simulink model "FG-fdm"  (R2022a)
settings: Solver=FixedStepAuto  StartTime=0.0  StopTime=Tend  FixedStep=Ts  MaxStep=0.033333333333333333  RelTol=1e-3
undefined symbols (not defined in the file or in its folder): A, B, C, D, Earth, h0, Ts, u0, v0, w0, WGS84, x0
libraries: aerolibconvert2 x3, aerolibfltsims x2, aerolibanimutils x1, aerolibtransform2 x1
settings Model: Creator=OSU  LastModifiedBy=Nick
settings DebuggingCC: UnconnectedInputMsg=warning  UnconnectedOutputMsg=warning  UnconnectedLineMsg=warning
settings RTWCC: DLArmComputeVersion=19.05

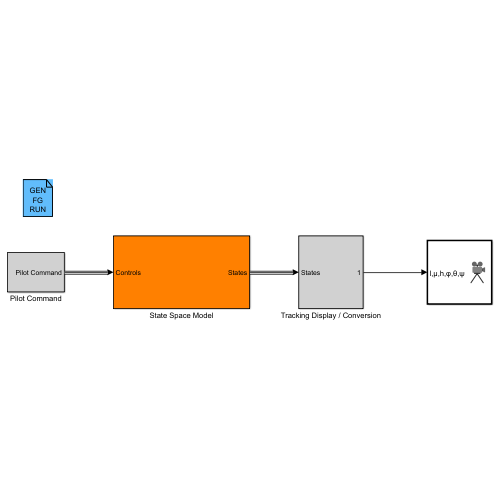
[thumbnail: Simulink's stored preview of the top-level diagram]
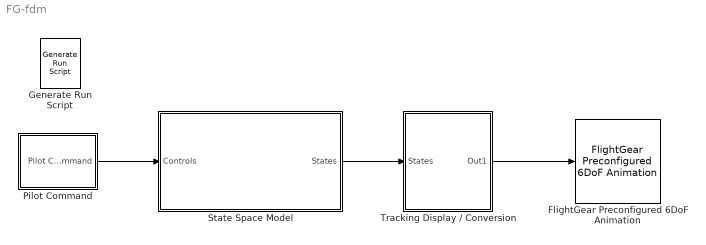
== system FG-fdm ==
  FlightGear Preconfigured 6DoF Animation : aerolibfltsims/FlightGear Preconfigured 6DoF Animation  xFlightGearVersion=v2019.1  DestinationIpAddress=127.0.0.1  DestinationPort=5502  SampleTime=Ts  packetVersion=24
  Generate Run Script : aerolibfltsims/Generate Run Script  Architecture=Default  dataFlow=Send  GeometryModelName=c172p_slx  AirportId=KSWO  RunwayId=35  InitialAltitude=5000  InitialHeading=0  OffsetDistance=0  OffsetAzimuth=0  InstallScenery=on  DisableShaders=off  OriginAddress=127.0.0.1  DestinationPort=5502  OriginPort=5505  LocalAddress=127.0.0.1  OutputFileName=runfg172p.bat  FlightGearBaseDirectory=C:\Program Files\FlightGear
  Pilot Command : Subsystem
  State Space Model : Subsystem
  Tracking Display / Conversion : Subsystem
  wires:
  Tracking Display / Conversion/1(Out1) -> FlightGear Preconfigured 6DoF Animation/1
  State Space Model/1(States) -> Tracking Display / Conversion/1(States)
  Pilot Command/1(Pilot Command) -> State Space Model/1(Controls)

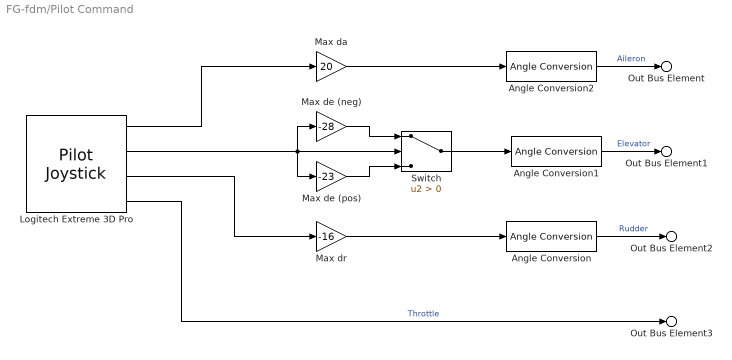
== system FG-fdm/Pilot Command ==
  Angle Conversion : aerolibconvert2/Angle Conversion  IU=deg  OU=rad
  Angle Conversion1 : aerolibconvert2/Angle Conversion  IU=deg  OU=rad
  Angle Conversion2 : aerolibconvert2/Angle Conversion  IU=deg  OU=rad
  Logitech Extreme 3D Pro : aerolibanimutils/Pilot Joystick  JoystickID=Joystick1  OutputConfiguration=FourAxis  SampleTime=Ts
  Max da : Gain  Gain=20
  Max de (neg) : Gain  Gain=-28
  Max de (pos) : Gain  Gain=-23
  Max dr : Gain  Gain=-16
  Switch : Switch  Criteria=u2 > Threshold  SaturateOnIntegerOverflow=off  InputSameDT=off
  Out Bus Element1 : Outport  PortName=Pilot Command  Element=Elevator
  Out Bus Element3 : Outport  PortName=Pilot Command  Element=Throttle
  Out Bus Element : Outport  PortName=Pilot Command  Element=Aileron
  Out Bus Element2 : Outport  PortName=Pilot Command  Element=Rudder
  wires:
  Logitech Extreme 3D Pro/3 -> Max dr/1
  Logitech Extreme 3D Pro/4 -> Out Bus Element3/1  "Throttle"
  Logitech Extreme 3D Pro/2 -> Max de (neg)/1, Max de (pos)/1, Switch/2
  Max de (neg)/1 -> Switch/1
  Max de (pos)/1 -> Switch/3
  Logitech Extreme 3D Pro/1 -> Max da/1
  Switch/1 -> Angle Conversion1/1
  Max da/1 -> Angle Conversion2/1
  Max dr/1 -> Angle Conversion/1
  Angle Conversion2/1 -> Out Bus Element/1  "Aileron"
  Angle Conversion1/1 -> Out Bus Element1/1  "Elevator"
  Angle Conversion/1 -> Out Bus Element2/1  "Rudder"

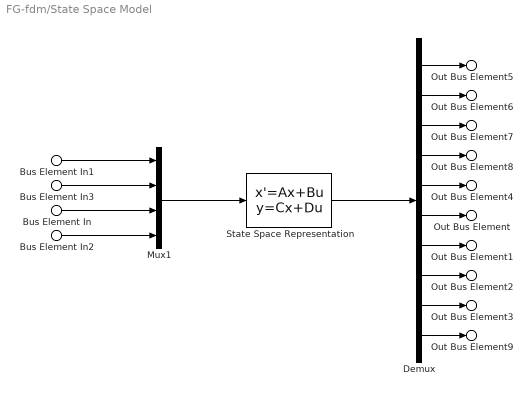
== system FG-fdm/State Space Model ==
  Bus Element In : Inport  PortName=Controls  Element=Aileron
  Bus Element In1 : Inport  PortName=Controls  Element=Elevator
  Bus Element In2 : Inport  PortName=Controls  Element=Rudder
  Bus Element In3 : Inport  PortName=Controls  Element=Throttle
  Demux : Demux  Outputs=10
  Mux1 : Mux
  State Space Representation : StateSpace  A=A  B=B  C=C  D=D  InitialCondition=x0
  Out Bus Element5 : Outport  PortName=States  Element=u
  Out Bus Element6 : Outport  PortName=States  Element=w
  Out Bus Element7 : Outport  PortName=States  Element=q
  Out Bus Element8 : Outport  PortName=States  Element=theta
  Out Bus Element : Outport  PortName=States  Element=v
  Out Bus Element1 : Outport  PortName=States  Element=p
  Out Bus Element2 : Outport  PortName=States  Element=r
  Out Bus Element3 : Outport  PortName=States  Element=phi
  Out Bus Element4 : Outport  PortName=States  Element=h
  Out Bus Element9 : Outport  PortName=States  Element=psi
  wires:
  Bus Element In/1 -> Mux1/3
  Bus Element In2/1 -> Mux1/4
  State Space Representation/1 -> Demux/1
  Demux/1 -> Out Bus Element5/1
  Demux/2 -> Out Bus Element6/1
  Demux/3 -> Out Bus Element7/1
  Demux/4 -> Out Bus Element8/1
  Bus Element In3/1 -> Mux1/2
  Mux1/1 -> State Space Representation/1
  Demux/5 -> Out Bus Element4/1
  Demux/6 -> Out Bus Element/1
  Demux/7 -> Out Bus Element1/1
  Demux/8 -> Out Bus Element2/1
  Demux/9 -> Out Bus Element3/1
  Demux/10 -> Out Bus Element9/1
  Bus Element In1/1 -> Mux1/1

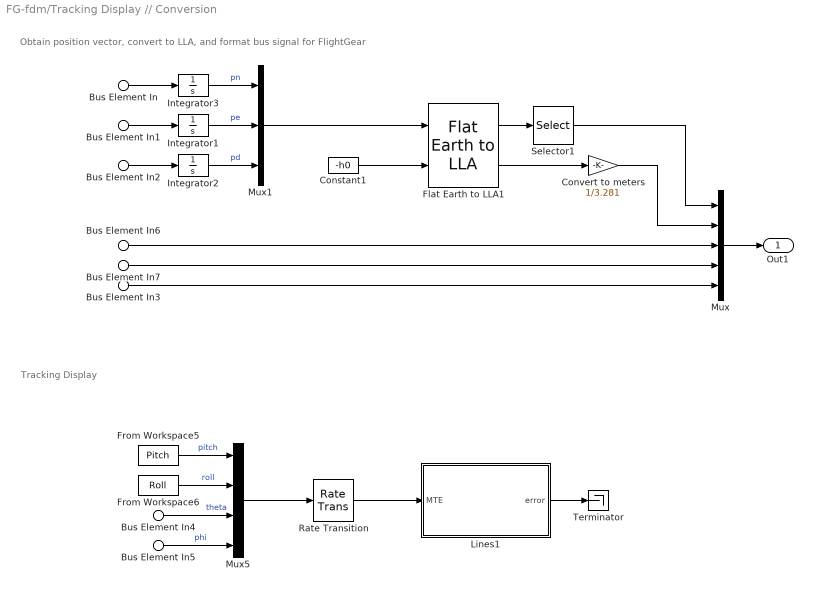
== system FG-fdm/Tracking Display // Conversion ==
  note: Tracking Display
  note: Obtain position vector, convert to LLA, and format bus signal for FlightGear
  Bus Element In : Inport  PortName=States  Element=u
  Bus Element In1 : Inport  PortName=States  Element=v
  Bus Element In2 : Inport  PortName=States  Element=w
  Bus Element In6 : Inport  PortName=States  Element=phi
  Bus Element In5 : Inport  PortName=States  Element=phi
  Bus Element In7 : Inport  PortName=States  Element=theta
  Bus Element In4 : Inport  PortName=States  Element=theta
  Bus Element In3 : Inport  PortName=States  Element=psi
  Constant1 : Constant  Value=-h0  SampleTime=Ts
  Convert to meters : Gain  Gain=1/3.281
  Flat Earth to LLA1 : aerolibtransform2/Flat Earth to LLA  units=English  ptype=Earth (WGS84)  F=1/298.257223563  R=20925646.3255  refPosPort=off  LL0=l_mu0  psi=0
  From Workspace5 : FromWorkspace  VariableName=Pitch  SampleTime=Ts  OutputAfterFinalValue=Setting to zero
  From Workspace6 : FromWorkspace  VariableName=Roll  SampleTime=Ts  OutputAfterFinalValue=Setting to zero
  Integrator1 : Integrator  InitialCondition=v0  ContinuousStateAttributes='v'
  Integrator2 : Integrator  InitialCondition=w0  ContinuousStateAttributes='w'
  Integrator3 : Integrator  InitialCondition=u0  ContinuousStateAttributes='u'
  Lines1 : MATLAB Function  TreatAsAtomicUnit=on
  Mux : Mux  Inputs=5
  Mux1 : Mux  Inputs=3
  Mux5 : Mux
  Rate Transition : RateTransition  OutPortSampleTimeOpt=Inherit  OutPortSampleTimeMultiple=2
  Selector1 : Selector  IndexMode=Zero-based  InputPortWidth=2  IndexOptions=Index vector (dialog)  Indices=[1 0]  OutputSizes=1
  Terminator : Terminator
  Out1 : Outport
  wires:
  Flat Earth to LLA1/1 -> Selector1/1
  Flat Earth to LLA1/2 -> Convert to meters/1
  Selector1/1 -> Mux/1
  Mux/1 -> Out1/1
  Bus Element In/1 -> Integrator3/1
  Bus Element In1/1 -> Integrator1/1
  Bus Element In6/1 -> Mux/3
  Bus Element In7/1 -> Mux/4
  Mux1/1 -> Flat Earth to LLA1/1
  Integrator1/1 -> Mux1/2  "pe"
  Integrator3/1 -> Mux1/1  "pn"
  Bus Element In2/1 -> Integrator2/1
  Bus Element In3/1 -> Mux/5
  Constant1/1 -> Flat Earth to LLA1/2
  Convert to meters/1 -> Mux/2
  Integrator2/1 -> Mux1/3  "pd"
  Bus Element In5/1 -> Mux5/4  "phi"
  Bus Element In4/1 -> Mux5/3  "theta"
  From Workspace6/1 -> Mux5/2  "roll"
  Mux5/1 -> Rate Transition/1
  From Workspace5/1 -> Mux5/1  "pitch"
  Lines1/1(error) -> Terminator/1
  Rate Transition/1 -> Lines1/1(MTE)

== matlab function FG-fdm/Tracking Display // Conversion/Lines1 ==
  data: MTE input; error output
function error = Display(MTE)

clf  % clear last frame

%-- Inputs --%
tht = MTE(1);
phi = MTE(2)*pi/180;
tht_x = MTE(3)*180/pi;
phi_x = MTE(4);

%-- Error signal output
error = [tht - tht_x; phi - phi_x];

%-- Transformation matrices --%
% MTE signal
R = [ cos(phi)  sin(phi)  0    ; 
     -sin(phi)  cos(phi) tht   ;
      0         0         1    ; ];
  
% Tolerance symbology
Rt = [ cos(phi_x)  sin(phi_x)  0     ;
      -sin(phi_x)  cos(phi_x)  tht_x ;
       0           0           1     ;];
   
    %% Calculate MTE signal and tolerance symbology orientation
        
%-- MTE signal line vector --%
% Transform vector coordinates
x0r = R * [ 10; 0; 1];     
x0l = R * [-10; 0; 1];

n = 25;     % for linspace()

% Transformed vector data for plotting
X = linspace(x0l(1), x0r(1), n);
Y = linspace(x0l(2), x0r(2), n);

%-- Tolerance vectors --%

% PITCH
rd = 1;     % Desired:  +/- 1 deg
ra = 2;     % Adequate: +/- 2 deg

ang = 0:0.01:2*pi;

xpd = rd*cos(ang);
ypd = rd*sin(ang);
xpa = ra*cos(ang);
ypa = ra*sin(ang);

N = ones(size(xpd));

Pd = Rt * [xpd; ypd; N];
Pa = Rt * [xpa; ypa; N];

% ROLL
td = 5*pi/180;     % Desired
ta = 10*pi/180;    % Adequate

% Define coordinates as vectors 
%      Top right  Bottom right  Top left   Bottom left
xRi = [ra*cos(td) ra*cos(-td) -ra*cos(td) -ra*cos(-td)...
       ra*cos(ta) ra*cos(-ta) -ra*cos(ta) -ra*cos(-ta);];
       
xRo = [10*cos(td) 10*cos(-td) -10*cos(td) -10*cos(-td)...
       10*cos(ta) 10*cos(-ta) -10*cos(ta) -10*cos(-ta);];

yRi = [ra*sin(td) ra*sin(-td) -ra*sin(td) -ra*sin(-td)...
       ra*sin(ta) ra*sin(-ta) -ra*sin(ta) -ra*sin(-ta);];
   
yRo = [10*sin(td) 10*sin(-td) -10*sin(td) -10*sin(-td)...
       10*sin(ta) 10*sin(-ta) -10*sin(ta) -10*sin(-ta);];

% Transform the coordinates 
Ri = Rt * [xRi; yRi; ones(size(xRi))];
Ro = Rt * [xRo; yRo; ones(size(xRo))];

% Generate vectors between transformed coordinates
XR = zeros(8, length(X));   % Preallocate storage
YR = zeros(8, length(X));

for i = 1:8
    XR(i, :) = linspace(Ri(1,i), Ro(1,i), n);
    YR(i, :) = linspace(Ri(2,i), Ro(2,i), n);
end


    %% Draw the transformed display
hold on
% axis equal
xlim([-20 20])
ylim([-20 20])
bgc = .25;
set(gca, 'Color', [bgc bgc bgc])

%- Draw tolerance -%
toc = 0.9;  % RGB color for light grey (tolerance color)

% PITCH
plot(Pd(1,:), Pd(2,:), 'Color', [toc toc toc], 'LineStyle', ':')
plot(Pa(1,:), Pa(2,:), 'Color', [toc toc toc], 'LineStyle','-.')

% ROLL
% Two loops for different LineStyle
for j = 1:4
    plot(XR(j,:), YR(j,:), 'Color', [toc toc toc], 'LineStyle',':')
end

for j = 5:8
    plot(XR(j,:), YR(j,:), 'Color', [toc toc toc], 'LineStyle','-.')
end


%- Draw MTE signal -%
plot(X, Y, 'Color', 'g')
plot(0, tht, 'Color', 'g','Marker','*')

hold off
drawnow

return
